simulink library "Counters_Lib"  (R2016a)
settings: Solver=ode45  StartTime=0.0  StopTime=10.0  RelTol=1e-3
libraries: simulink_extras x16
settings Model: Creator=Jozko Mrkvicka  LastModifiedBy=Jozko Mrkvicka
settings DataIOCC: LimitDataPoints=on
settings DebuggingCC: AllowSymbolicDim=off

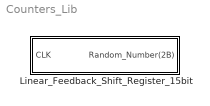
== system Counters_Lib ==
  Linear_Feedback_Shift_Register_15bit : Subsystem

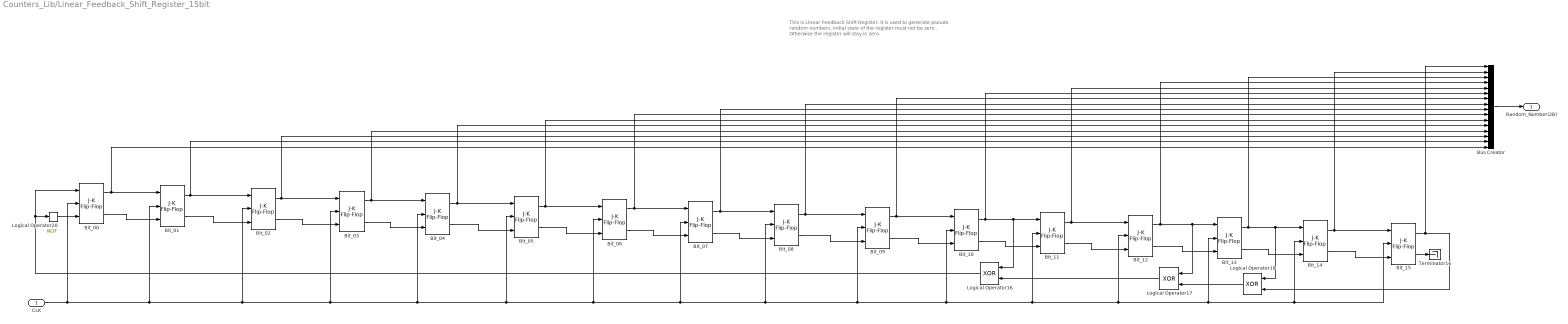
== system Counters_Lib/Linear_Feedback_Shift_Register_15bit ==
  note: This is Linear Feedback Shift Register. It is used to generate pseudo random numbers. Initial state of the register must not be zero . Otherwise the register will stay in zero.
  CLK : Inport
  Bit_00 : simulink_extras/Flip Flops/J-K Flip-Flop  initial_condition=1
  Bit_01 : simulink_extras/Flip Flops/J-K Flip-Flop  initial_condition=0
  Bit_02 : simulink_extras/Flip Flops/J-K Flip-Flop  initial_condition=0
  Bit_03 : simulink_extras/Flip Flops/J-K Flip-Flop  initial_condition=0
  Bit_04 : simulink_extras/Flip Flops/J-K Flip-Flop  initial_condition=0
  Bit_05 : simulink_extras/Flip Flops/J-K Flip-Flop  initial_condition=0
  Bit_06 : simulink_extras/Flip Flops/J-K Flip-Flop  initial_condition=0
  Bit_07 : simulink_extras/Flip Flops/J-K Flip-Flop  initial_condition=0
  Bit_08 : simulink_extras/Flip Flops/J-K Flip-Flop  initial_condition=0
  Bit_09 : simulink_extras/Flip Flops/J-K Flip-Flop  initial_condition=0
  Bit_{10..15} (6 alike) : simulink_extras/Flip Flops/J-K Flip-Flop  initial_condition=0
  Bus Creator : BusCreator  Inputs=16
  Logical Operator16 : Logic  Operator=XOR  IconShape=distinctive  AllPortsSameDT=off  OutDataTypeStr=boolean
  Logical Operator17 : Logic  Operator=XOR  IconShape=distinctive  AllPortsSameDT=off  OutDataTypeStr=boolean
  Logical Operator18 : Logic  Operator=XOR  IconShape=distinctive  AllPortsSameDT=off  OutDataTypeStr=boolean
  Logical Operator20 : Logic  Operator=NOT  IconShape=distinctive  AllPortsSameDT=off  OutDataTypeStr=boolean
  Terminator16 : Terminator
  Random_Number(2B) : Outport
  wires:
  Logical Operator20/1 -> Bit_00/3
  Bit_14/2 -> Bit_15/3
  Bit_06/2 -> Bit_07/3
  Bit_04/2 -> Bit_05/3
  Logical Operator18/1 -> Logical Operator17/2
  Logical Operator17/1 -> Logical Operator16/2
  Bit_00/2 -> Bit_01/3
  Logical Operator16/1 -> Logical Operator20/1, Bit_00/1
  Bit_02/2 -> Bit_03/3
  Bit_03/2 -> Bit_04/3
  Bit_01/2 -> Bit_02/3
  Bit_05/2 -> Bit_06/3
  Bit_07/2 -> Bit_08/3
  Bit_09/2 -> Bit_10/3
  Bit_10/2 -> Bit_11/3
  Bit_08/2 -> Bit_09/3
  Bit_13/2 -> Bit_14/3
  Bit_12/2 -> Bit_13/3
  Bit_11/2 -> Bit_12/3
  Bit_00/1 -> Bus Creator/16, Bit_01/1
  CLK/1 -> Bit_00/2, Bit_01/2, Bit_02/2, Bit_03/2, Bit_04/2, Bit_05/2, Bit_06/2, Bit_07/2, Bit_08/2, Bit_09/2, Bit_10/2, Bit_11/2, Bit_12/2, Bit_13/2, Bit_14/2, Bit_15/2
  Bit_15/1 -> Bus Creator/1, Logical Operator18/2
  Bit_15/2 -> Terminator16/1
  Bit_01/1 -> Bus Creator/15, Bit_02/1
  Bit_02/1 -> Bus Creator/14, Bit_03/1
  Bit_03/1 -> Bus Creator/13, Bit_04/1
  Bit_04/1 -> Bus Creator/12, Bit_05/1
  Bit_05/1 -> Bus Creator/11, Bit_06/1
  Bit_06/1 -> Bus Creator/10, Bit_07/1
  Bit_07/1 -> Bus Creator/9, Bit_08/1
  Bit_08/1 -> Bus Creator/8, Bit_09/1
  Bit_09/1 -> Bus Creator/7, Bit_10/1
  Bit_10/1 -> Bus Creator/6, Bit_11/1, Logical Operator16/1
  Bit_12/1 -> Bus Creator/4, Bit_13/1, Logical Operator17/1
  Bit_13/1 -> Bus Creator/3, Bit_14/1, Logical Operator18/1
  Bit_14/1 -> Bus Creator/2, Bit_15/1
  Bit_11/1 -> Bus Creator/5, Bit_12/1
  Bus Creator/1 -> Random_Number(2B)/1
